simulink model "kalmanFilter"  (R2023b)
settings: Solver=FixedStepAuto  StartTime=0.0  StopTime=Tfinal  FixedStep=dt_KF  RelTol=1e-3
model workspace (MAT data in the model file):
  P0 = [0.001  0  0  0  0  0; 0  0.001  0  0  0  0; 0  0  0.001  0  0  0; 0  0  0  0.001  0  0; 0  0  0  0  0.001  0; 0  0  0  0  0  0.001]
  Q = [1e-05  0  0  0  0  0; 0  1e-05  0  0  0  0; 0  0  1e-05  0  0  0; 0  0  0  1e-05  0  0; 0  0  0  0  1e-05  0; 0  0  0  0  0  1e-05]
  R = [1 0 0 0 0 0 0 0 0 0 0 0 ... (1296 elements, 36x36)]
  dt_KF = 1
libraries: rotationConversionLib x2, matrix_library x1
settings Model: Creator=kristopherriordan  LastModifiedBy=kristopherriordan

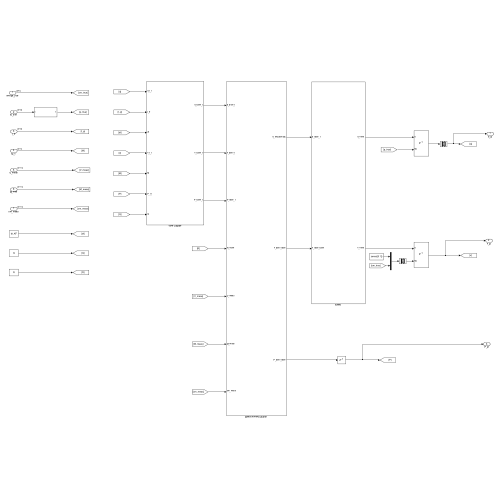
[thumbnail: Simulink's stored preview of the top-level diagram]
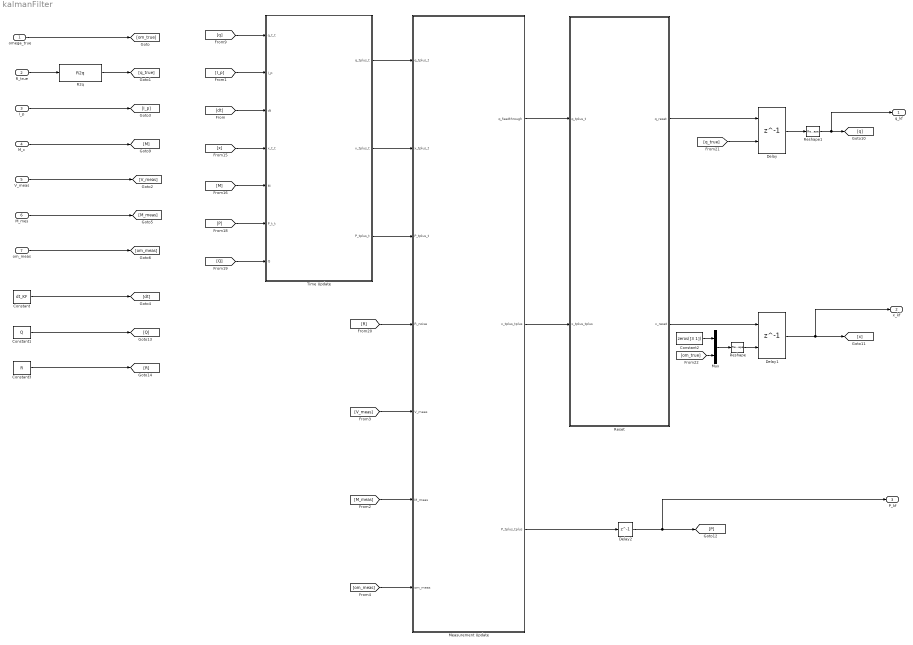
== system kalmanFilter ==
  omega_true : Inport  PortDimensions=[3 1]
  R_true : Inport  Port=2  PortDimensions=[3 3]
  I_p : Inport  Port=3  PortDimensions=[3 3]
  M_c : Inport  Port=4  PortDimensions=[3 1]
  V_meas : Inport  Port=5  PortDimensions=[3 11]
  M_mes : Inport  Port=6  PortDimensions=[3 11]
  om_meas : Inport  Port=7  PortDimensions=[3 11]
  Constant : Constant  Value=dt_KF
  Constant1 : Constant  Value=Q
  Constant2 : Constant  Value=zeros([3 1])
  Constant3 : Constant  Value=R
  Delay : Delay  DelayLength=1  InitialConditionSource=Input port  InitialCondition=0
      settings: InputPortMap=u0,p4
  Delay1 : Delay  DelayLength=1  InitialConditionSource=Input port  InitialCondition=0
      settings: InputPortMap=u0,p4
  Delay2 : Delay  DelayLength=1  InitialCondition=P0
  "Measurement Update " : Subsystem
  Mux : Mux  Inputs=2
  R2q : rotationConversionLib/R2q  SystemSampleTime=-1  VariantActivationTime=update diagram  AllowFlexibleInterface=on  Latency=0  AutoFrameSizeCalculation=off
  Reset : Subsystem
  Reshape : Reshape  OutputDimensionality=Column vector (2-D)
  Reshape1 : Reshape  OutputDimensionality=Column vector (2-D)
  Time Update : Subsystem
  q_kf : Outport
  x_kf : Outport  Port=2
  P_kf : Outport  Port=3
  wires:
  R_true/1 -> R2q/1
  omega_true/1 -> [om_true]
  R2q/1 -> [q_true]
  Constant/1 -> [dt]
  I_p/1 -> [I_p]
  [q] -> Time Update/1(q_t_t)
  [x] -> Time Update/4(x_t_t)
  M_c/1 -> [M]
  [M] -> Time Update/5(M)
  Time Update/1(q_tplus_t) -> "Measurement Update "/1(q_tplus_t)
  Time Update/2(x_tplus_t) -> "Measurement Update "/2(x_tplus_t)
  "Measurement Update "/1(q_feedthrough) -> Reset/1(q_tplus_t)
  "Measurement Update "/2(x_tplus_tplus) -> Reset/2(x_tplus_tplus)
  Reset/1(q_reset) -> Delay/1
  Reset/2(x_reset) -> Delay1/1
  Delay/1 -> Reshape1/1
  Time Update/3(P_tplus_t) -> "Measurement Update "/3(P_tplus_t)
  Delay1/1 -> x_kf/1, [x]
  "Measurement Update "/3(P_tplus_tplus) -> Delay2/1
  Delay2/1 -> P_kf/1, [P]
  [P] -> Time Update/6(P_t_t)
  Constant1/1 -> [Q]
  [Q] -> Time Update/7(Q)
  Constant3/1 -> [R]
  [R] -> "Measurement Update "/4(R_noise)
  [q_true] -> Delay/2
  Reshape/1 -> Delay1/2
  Mux/1 -> Reshape/1
  [om_true] -> Mux/2
  Constant2/1 -> Mux/1
  [I_p] -> Time Update/2(I_p)
  [dt] -> Time Update/3(dt)
  Reshape1/1 -> q_kf/1, [q]
  V_meas/1 -> [V_meas]
  M_mes/1 -> [M_meas]
  om_meas/1 -> [om_meas]
  [V_meas] -> "Measurement Update "/5(V_meas)
  [M_meas] -> "Measurement Update "/6(M_meas)
  [om_meas] -> "Measurement Update "/7(om_meas)

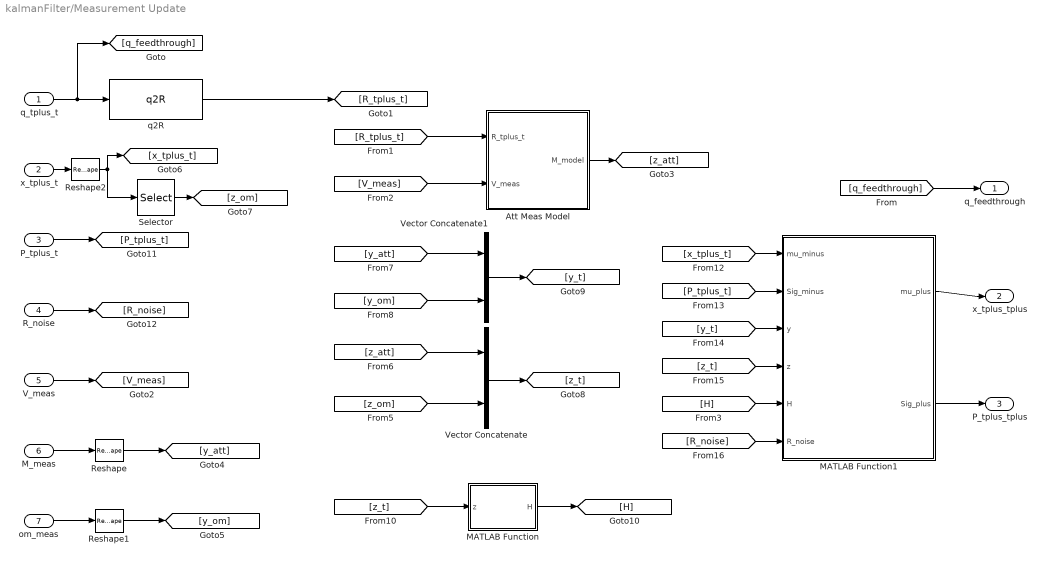
== system kalmanFilter/Measurement Update  ==
  q_tplus_t : Inport
  x_tplus_t : Inport  Port=2
  P_tplus_t : Inport  Port=3
  R_noise : Inport  Port=4
  V_meas : Inport  Port=5
  M_meas : Inport  Port=6
  om_meas : Inport  Port=7
  Att Meas Model : Subsystem
  MATLAB Function : MATLAB Function  TreatAsAtomicUnit=on
  MATLAB Function1 : MATLAB Function  TreatAsAtomicUnit=on
  Reshape : Reshape  OutputDimensionality=Column vector (2-D)
  Reshape1 : Reshape  OutputDimensionality=Column vector (2-D)
  Reshape2 : Reshape  OutputDimensionality=Column vector (2-D)
  Selector : Selector  NumberOfDimensions=2  InputPortWidth=3  IndexOptions=Index vector (dialog),Index vector (dialog)  Indices=[4:6],1  OutputSizes=1,1
  Vector Concatenate : Concatenate
  Vector Concatenate1 : Concatenate
  q2R : rotationConversionLib/q2R  SystemSampleTime=-1  VariantActivationTime=update diagram  AllowFlexibleInterface=on  Latency=0  AutoFrameSizeCalculation=off
  q_feedthrough : Outport
  x_tplus_tplus : Outport  Port=2
  P_tplus_tplus : Outport  Port=3
  wires:
  q_tplus_t/1 -> [q_feedthrough], q2R/1
  R_noise/1 -> [R_noise]
  [q_feedthrough] -> q_feedthrough/1
  q2R/1 -> [R_tplus_t]
  [R_tplus_t] -> Att Meas Model/1(R_tplus_t)
  [V_meas] -> Att Meas Model/2(V_meas)
  V_meas/1 -> [V_meas]
  Att Meas Model/1(M_model) -> [z_att]
  M_meas/1 -> Reshape/1
  Reshape/1 -> [y_att]
  om_meas/1 -> Reshape1/1
  Reshape1/1 -> [y_om]
  Selector/1 -> [z_om]
  Reshape2/1 -> Selector/1, [x_tplus_t]
  x_tplus_t/1 -> Reshape2/1
  [z_att] -> Vector Concatenate/1
  [z_om] -> Vector Concatenate/2
  Vector Concatenate/1 -> [z_t]
  [y_att] -> Vector Concatenate1/1
  [y_om] -> Vector Concatenate1/2
  Vector Concatenate1/1 -> [y_t]
  [z_t] -> MATLAB Function/1(z)
  MATLAB Function/1(H) -> [H]
  [x_tplus_t] -> MATLAB Function1/1(mu_minus)
  [P_tplus_t] -> MATLAB Function1/2(Sig_minus)
  P_tplus_t/1 -> [P_tplus_t]
  [y_t] -> MATLAB Function1/3(y)
  [z_t] -> MATLAB Function1/4(z)
  [R_noise] -> MATLAB Function1/6(R_noise)
  MATLAB Function1/2(Sig_plus) -> P_tplus_tplus/1
  MATLAB Function1/1(mu_plus) -> x_tplus_tplus/1
  [H] -> MATLAB Function1/5(H)

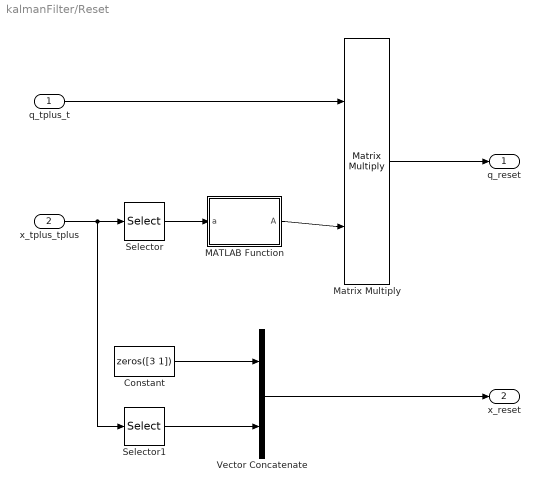
== system kalmanFilter/Reset ==
  q_tplus_t : Inport
  x_tplus_tplus : Inport  Port=2
  Constant : Constant  Value=zeros([3 1])  VectorParams1D=off
  MATLAB Function : MATLAB Function  TreatAsAtomicUnit=on
  Matrix Multiply : Product  Multiplication=Matrix(*)
  Selector : Selector  NumberOfDimensions=2  InputPortWidth=3  IndexOptions=Index vector (dialog),Index vector (dialog)  Indices=[1:3],1  OutputSizes=1,1
  Selector1 : Selector  NumberOfDimensions=2  InputPortWidth=3  IndexOptions=Index vector (dialog),Index vector (dialog)  Indices=[4:6],1  OutputSizes=1,1
  Vector Concatenate : Concatenate
  q_reset : Outport
  x_reset : Outport  Port=2
  wires:
  q_tplus_t/1 -> Matrix Multiply/1
  x_tplus_tplus/1 -> Selector1/1, Selector/1
  Selector/1 -> MATLAB Function/1(a)
  MATLAB Function/1(A) -> Matrix Multiply/2
  Matrix Multiply/1 -> q_reset/1
  Selector1/1 -> Vector Concatenate/2
  Constant/1 -> Vector Concatenate/1
  Vector Concatenate/1 -> x_reset/1

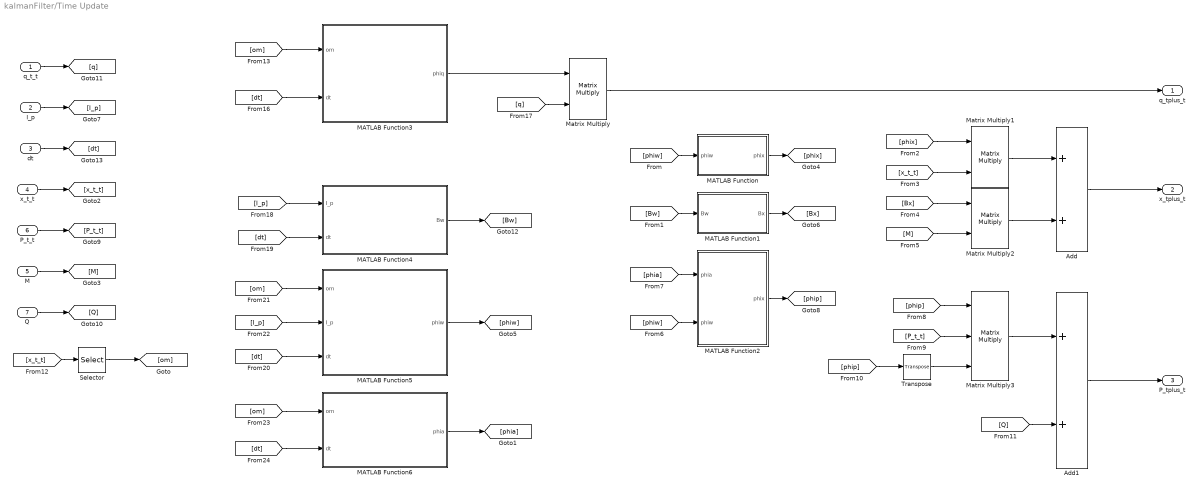
== system kalmanFilter/Time Update ==
  q_t_t : Inport
  I_p : Inport  Port=2
  dt : Inport  Port=3
  x_t_t : Inport  Port=4
  M : Inport  Port=5
  P_t_t : Inport  Port=6
  Q : Inport  Port=7
  Add : Sum
  Add1 : Sum
  MATLAB Function : MATLAB Function  TreatAsAtomicUnit=on
  MATLAB Function1 : MATLAB Function  TreatAsAtomicUnit=on
  MATLAB Function2 : MATLAB Function  TreatAsAtomicUnit=on
  MATLAB Function3 : MATLAB Function  TreatAsAtomicUnit=on
  MATLAB Function4 : MATLAB Function  TreatAsAtomicUnit=on
  MATLAB Function5 : MATLAB Function  TreatAsAtomicUnit=on
  MATLAB Function6 : MATLAB Function  TreatAsAtomicUnit=on
  Matrix Multiply : Product  Multiplication=Matrix(*)
  Matrix Multiply1 : Product  Multiplication=Matrix(*)
  Matrix Multiply2 : Product  Multiplication=Matrix(*)
  Matrix Multiply3 : Product  Inputs=***  Multiplication=Matrix(*)
  Selector : Selector  NumberOfDimensions=2  InputPortWidth=3  IndexOptions=Index vector (dialog),Index vector (dialog)  Indices=[4:6],1  OutputSizes=1,1
  Transpose : matrix_library/Transpose
  q_tplus_t : Outport
  x_tplus_t : Outport  Port=2
  P_tplus_t : Outport  Port=3
  wires:
  MATLAB Function3/1(phiq) -> Matrix Multiply/1
  Matrix Multiply/1 -> q_tplus_t/1
  x_t_t/1 -> [x_t_t]
  M/1 -> [M]
  [phiw] -> MATLAB Function/1(phiw)
  [Bw] -> MATLAB Function1/1(Bw)
  MATLAB Function/1(phix) -> [phix]
  MATLAB Function1/1(Bx) -> [Bx]
  [phix] -> Matrix Multiply1/1
  [x_t_t] -> Matrix Multiply1/2
  [Bx] -> Matrix Multiply2/1
  [M] -> Matrix Multiply2/2
  Matrix Multiply1/1 -> Add/1
  Matrix Multiply2/1 -> Add/2
  Add/1 -> x_tplus_t/1
  [phiw] -> MATLAB Function2/2(phiw)
  [phia] -> MATLAB Function2/1(phia)
  MATLAB Function2/1(phix) -> [phip]
  P_t_t/1 -> [P_t_t]
  [phip] -> Matrix Multiply3/1
  [P_t_t] -> Matrix Multiply3/2
  Transpose/1 -> Matrix Multiply3/3
  [phip] -> Transpose/1
  Matrix Multiply3/1 -> Add1/1
  Q/1 -> [Q]
  [Q] -> Add1/2
  Add1/1 -> P_tplus_t/1
  [x_t_t] -> Selector/1
  Selector/1 -> [om]
  [om] -> MATLAB Function3/1(om)
  q_t_t/1 -> [q]
  [dt] -> MATLAB Function3/2(dt)
  [q] -> Matrix Multiply/2
  MATLAB Function4/1(Bw) -> [Bw]
  [I_p] -> MATLAB Function4/1(I_p)
  [dt] -> MATLAB Function4/2(dt)
  [om] -> MATLAB Function5/1(om)
  MATLAB Function5/1(phiw) -> [phiw]
  [dt] -> MATLAB Function5/3(dt)
  [I_p] -> MATLAB Function5/2(I_p)
  [dt] -> MATLAB Function6/2(dt)
  MATLAB Function6/1(phia) -> [phia]
  [om] -> MATLAB Function6/1(om)
  I_p/1 -> [I_p]
  dt/1 -> [dt]

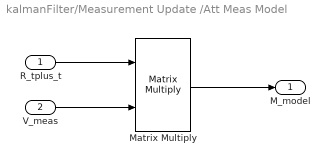
== system kalmanFilter/Measurement Update /Att Meas Model ==
  R_tplus_t : Inport
  V_meas : Inport  Port=2
  Matrix Multiply : Product  Multiplication=Matrix(*)
  M_model : Outport
  wires:
  V_meas/1 -> Matrix Multiply/2
  R_tplus_t/1 -> Matrix Multiply/1
  Matrix Multiply/1 -> M_model/1

== matlab function kalmanFilter/Measurement Update /MATLAB Function1 ==
  data: mu_minus input; mu_plus output; Sig_minus input; y input; z input; H input; R_noise input; Sig_plus output
function [mu_plus, Sig_plus] = measUpdate(mu_minus, Sig_minus, y, z, H, R_noise)

K = (Sig_minus * H.')\(H * Sig_minus * H.' + R_noise);

mu_plus = mu_minus + K * (y - z);
Sig_plus = Sig_minus - K * H * Sig_minus;

== matlab function kalmanFilter/Measurement Update /MATLAB Function ==
  data: z input; H output
function H = constructH(z)

z_att = z(:,end-3);
% z_om = z(end-2:end);

n = uint32(length(z_att));

H_att = zeros([3, 3*n]);

iters = n/3;

for i=1:iters
    H_att(:, (3*(i-1) + 1):(3*(i-1) + 1 + 2)) = vcross( z( (3*(i-1) + 1):(3*(i-1) + 1 + 2) ) );
end

H = [H_att.', zeros(size(H_att.'));
    zeros([3 3]), eye(3)];

    function V = vcross(v)
        V = [0, -v(3), v(2);
            v(3), 0, -v(1);
            -v(2), v(1), 0];
    end

end

== matlab function kalmanFilter/Reset/MATLAB Function ==
  data: a input; A output
function A = constructA(a)

ax = a(1);
ay = a(2);
az = a(3);

A = eye(4) + (1/2).*[0, -ax, -ay, -az;
                    ax, 0, ax, -ay;
                    ay, -az, 0, ax;
                    az, ay, -ax, 0];

== matlab function kalmanFilter/Time Update/MATLAB Function ==
  data: phiw input; phix output
function phix = constructPhiX(phiw)

phix = [eye(3), zeros([3 3]);
        zeros([3 3]), phiw];

== matlab function kalmanFilter/Time Update/MATLAB Function1 ==
  data: Bw input; Bx output
function Bx = constructBx(Bw)

Bx = [zeros([3 3]);
      Bw];

== matlab function kalmanFilter/Time Update/MATLAB Function2 ==
  data: phia input; phiw input; phix output
function phix = constructPhiX(phia, phiw)

phix = [phia, zeros([3 3]);
        zeros([3 3]), phiw];

== matlab function kalmanFilter/Time Update/MATLAB Function3 ==
  data: om input size=[3 1]; phiq output double size=[4 4]; dt input
function phiq = constructPhiQ(om, dt)

om1 = om(1);
om2 = om(2);
om3 = om(3);
ommag = norm(om);

% q0 = q(1);
% q1 = q(2);
% q2 = q(3);
% q3 = q(4);

% Ixyz = diag(I_p);
% Ix = Ixyz(1);
% Iy = Ixyz(2);
% Iz = Ixyz(3);

C = cos(ommag*dt/2);
S = (1/(ommag + 1e-10))*sin(ommag*dt/2);

% phiw = [1, (Iy - Iz)*om3/Ix, (Iy-Iz)*om2/Ix;
        % (Iz - Ix)*om3/Iy, 1, (Iz - Ix)*om1/Iy;
        % (Ix - Iy)*om2/Iz, (Ix - Iy)*om1/Iz, 1];

phiq = [C, -S*om1, -S*om2, -S*om3;
        S*om1, C, S*om3, -S*om2;
        S*om2, -S*om3, C, S*om1;
        S*om3, S*om2, -S*om1, C];

% phi = [phiw, zeros([3 4]);phiq];

== matlab function kalmanFilter/Time Update/MATLAB Function4 ==
  data: I_p input; Bw output; dt input
function Bw = constructBw(I_p, dt)

Ixyz = diag(I_p);
Ix = Ixyz(1);
Iy = Ixyz(2);
Iz = Ixyz(3);

Bw = dt.*[1/Ix, 0, 0;
          0, 1/Iy, 0;
          0, 0, 1/Iz];

% B = [Bw;zeros([4 3])];

== matlab function kalmanFilter/Time Update/MATLAB Function5 ==
  data: om input; phiw output; I_p input; dt input
function phiw = consructPhiOm(om, I_p, dt)

Ixyz = diag(I_p);
Ix = Ixyz(1);
Iy = Ixyz(2);
Iz = Ixyz(3);

om1 = om(1);
om2 = om(2);
om3 = om(3);


phiw = eye(3) + (dt/2).*[0, (Iy - Iz)*om3/Ix, (Iy-Iz)*om2/Ix;
                (Iz - Ix)*om3/Iy, 0, (Iz - Ix)*om1/Iy;
                (Ix - Iy)*om2/Iz, (Ix - Iy)*om1/Iz, 0];

== matlab function kalmanFilter/Time Update/MATLAB Function6 ==
  data: om input; phia output size=[3 3]; dt input
function phia = constructPhiA(om, dt)

om1 = om(1);
om2 = om(2);
om3 = om(3);

omcross = [0 -om3 om2;
           om3 0 -om1;
           -om2 om1 0];

ommag = norm(om);

C = cos(ommag*dt/2);
S = (1/(ommag + 1e-10))*sin(ommag*dt/2);

phia = eye(3) + S.*omcross + ((1 - C)/ommag^2).*(omcross*omcross);
